simulink model "TestModel"  (R2023a)
settings: Solver=VariableStepAuto  StartTime=0.0  StopTime=10.0  RelTol=1e-3
settings Model: Creator=jack2  LastModifiedBy=jack2

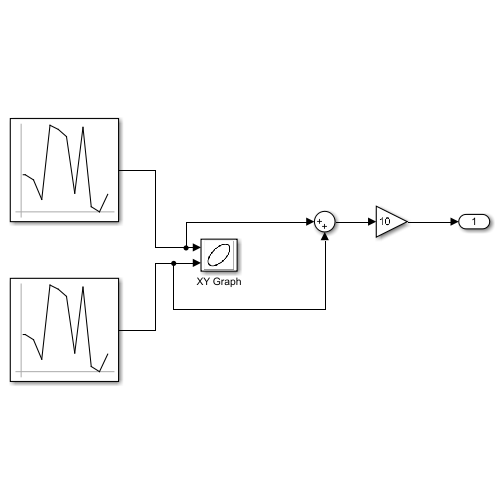
[thumbnail: Simulink's stored preview of the top-level diagram]
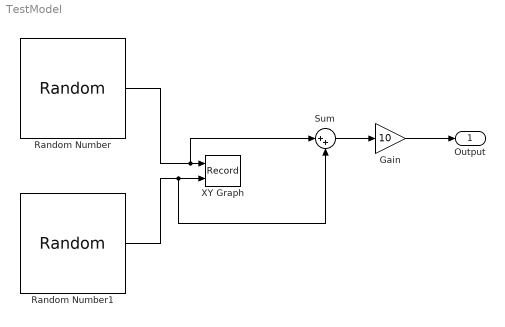
== system TestModel ==
  Gain : Gain  Gain=10
  Random Number : RandomNumber  Seed=1  SampleTime=0.1
  Random Number1 : RandomNumber  Seed=2  SampleTime=0.1
  Sum : Sum  Inputs=|++
  XY Graph : Record  FileSettingsInternal="{\"entries\":[{\"content\":{\"excelSettings\":{\"content\":{},\"type\":\"Streamout.ExcelSettings\"}},\"type\":\"Streamout.FileSettingStorage\",\"uuid\":\"1e30b135-2edb-46c3-8150-21f8e321084e\"}],\"packageUris\":[\"http://schema.mathworks.com/mf0/streamout_blocks/R2020a\"],\"version\":\"1.0\"}"  Layout=[1 1]  SignalsInternal="{\"entries\":[{\"content\":{\"signals\":[{\"content\":{\"blockPath\":[\"TestModel/XY Graph\"],\"dimensions\":[1],\"domain\":\"TestModel/XY Graph\",\"lineColor\":\"#a2142f\",\"plots\":[1],\"port\":1,\"sid\":[\"\"],\"signalID\":33,\"signalName\":\"Random\\nNumber\"},\"type\":\"RecordBlkView.Signal\",\"uuid\":\"adc23962-0999-4655-8133-462975201274\"},{\"content\":{\"blockPath\":[\"TestModel/XY Graph\"],\"dimensions\":[1],\"domain\":\"TestModel/XY Graph\",\"lineColor\":\"#139fff\",\"plots\":[1],\"port\":2,\"sid\":[\"\"],\"signalID\":37,\"signalName\":\"Random\\nNumber1\"},\"type\":\"RecordBlkView.Signal\",\"uuid\":\"cc444ba0-aa5f-47e9-81b9-fafe2dbe71b8\"}]},\"type\":\"RecordBlkView.InputSignals\",\"uuid\":\"aab05ad6-6780-4906-8000-e6d313b2030e\"}],\"packageUris\":[\"http://schema.mathworks.com/mf0/streamout_blocks/R2020a\"],\"version\":\"1.0\"}"  VisualizationBindings="{\"xyplotplugin\":{\"info\":[{\"series\":[{\"bindingParametersList\":[{\"parameter\":\"X-Axis\",\"signalID\":33,\"signalName\":\"Random\\nNumber\"},{\"parameter\":\"Y-Axis\",\"signalID\":37,\"signalName\":\"Random\\nNumber1\"}],\"seriesID\":6963}],\"subplotID\":1}]}}"  CompatibilityTag=XY
  Output : Outport
  wires:
  Random Number/1 -> Sum/1, XY Graph/1
  Random Number1/1 -> Sum/2, XY Graph/2
  Sum/1 -> Gain/1
  Gain/1 -> Output/1
